simulink model "PIDnLQR"  (R2021a)
settings: Solver=VariableStepAuto  StartTime=0.0  StopTime=4500  RelTol=1e-3
values from neighbouring files (symbols this model uses):
  FF = 1/y(end)    [main.m]
  M = c2d(Mcon,Ts,'zoh')    [main.m]
  SYSdaug = ss(Aaug,Baug,Caug,[],Ts)    [main.m]
  Ts = Mrise/15    [main.m]
undefined symbols (not defined in the file or in its folder): Klqr
libraries: pid_lib x1
settings Model: Creator=andre  LastModifiedBy=Nidhin
settings SolverCC: AlgebraicLoopSolver=TrustRegion
settings DebuggingCC: SFMachineParentedDataDiag=warning

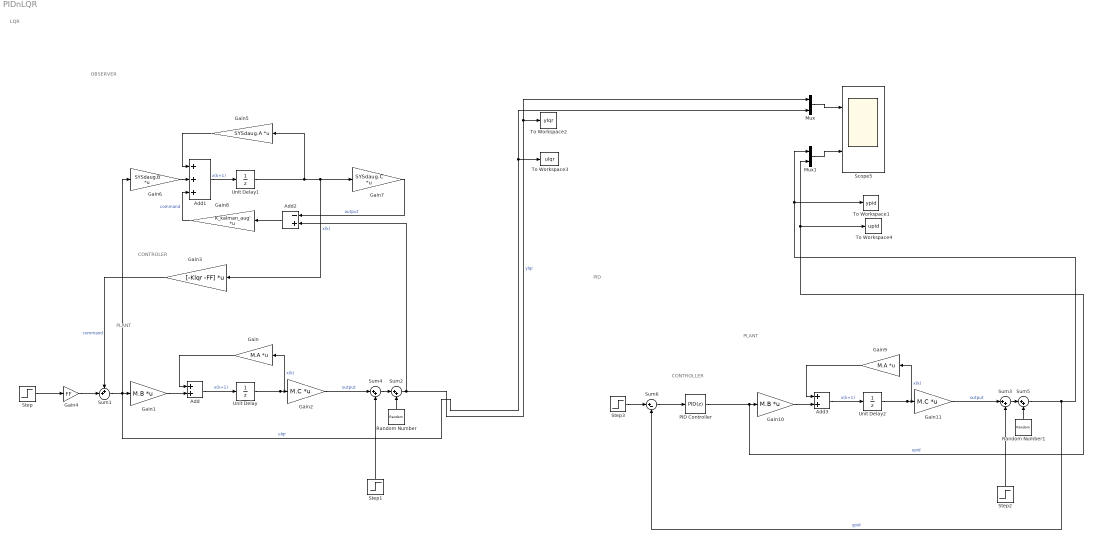
== system PIDnLQR ==
  note: PID
  note: CONTROLLER
  note: CONTROLER
  note: OBSERVER
  note: PLANT
  note: PLANT
  note: LQR
  Add : Sum
  Add1 : Sum  Inputs=+++
  Add2 : Sum  Inputs=-+
  Add3 : Sum
  Gain : Gain  Gain=M.A  Multiplication=Matrix(K*u)
  Gain1 : Gain  Gain=M.B  Multiplication=Matrix(K*u)
  Gain10 : Gain  Gain=M.B  Multiplication=Matrix(K*u)
  Gain11 : Gain  Gain=M.C  Multiplication=Matrix(K*u)
  Gain2 : Gain  Gain=M.C  Multiplication=Matrix(K*u)
  Gain3 : Gain  Gain=[-Klqr -FF]  Multiplication=Matrix(K*u)
  Gain4 : Gain  Gain=FF
  Gain5 : Gain  Gain=SYSdaug.A  Multiplication=Matrix(K*u)
  Gain6 : Gain  Gain=SYSdaug.B  Multiplication=Matrix(K*u)
  Gain7 : Gain  Gain=SYSdaug.C  Multiplication=Matrix(K*u)
  Gain8 : Gain  Gain=K_kalman_aug'  Multiplication=Matrix(K*u)
  Gain9 : Gain  Gain=M.A  Multiplication=Matrix(K*u)
  Mux : Mux  Inputs=2
  Mux1 : Mux  Inputs=2
  PID Controller : pid_lib/PID Controller  Controller=PID  Form=Parallel  TimeDomain=Discrete-time  UseExternalTs=off  SampleTime=Ts  IntegratorMethod=Forward Euler  FilterMethod=Forward Euler  ControllerParametersSource=internal  P=0.051105898923896  I=0.00228966428482342  D=0  UseFilter=on  N=100  TunerSelectOption=Transfer Function Based (PID Tuner App)  InitialConditionSource=internal  InitialConditionForIntegrator=0  InitialConditionForFilter=0  DifferentiatorICPrevScaledInput=0  ExternalReset=none  TrackingMode=off  Kt=1  LimitOutput=off  SatLimitsSource=internal  UpperSaturationLimit=inf  LowerSaturationLimit=-inf  LinearizeAsGain=on  AntiWindupMode=none  Kb=1  POutMin=[]  POutMax=[]  IOutMin=[]  IOutMax=[]  DOutMin=[]  DOutMax=[]  NOutMin=[]  NOutMax=[]  SumOutMin=[]  SumOutMax=[]  SaturationOutMin=[]  SaturationOutMax=[]  PParamMin=[]  PParamMax=[]  IParamMin=[]  IParamMax=[]  DParamMin=[]  DParamMax=[]  NParamMin=[]  NParamMax=[]  KbParamMin=[]  KbParamMax=[]  KtParamMin=[]  KtParamMax=[]  KbOutMin=[]  KbOutMax=[]  KtOutMin=[]  KtOutMax=[]  IntegratorOutMin=[]  IntegratorOutMax=[]  FilterOutMin=[]  FilterOutMax=[]  SumI1OutMin=[]  SumI1OutMax=[]  SumI2OutMin=[]  SumI2OutMax=[]  SumI3OutMin=[]  SumI3OutMax=[]  SumI4OutMin=[]  SumI4OutMax=[]  SumDOutMin=[]  SumDOutMax=[]  DifferentiatorOutMin=[]  DifferentiatorOutMax=[]  FilterDiffOutCoefMin=[]  FilterDiffOutCoefMax=[]  ReciprocalOutMin=[]  ReciprocalOutMax=[]  SumDenOutMin=[]  SumDenOutMax=[]  SumNumOutMin=[]  SumNumOutMax=[]  DivideOutMin=[]  DivideOutMax=[]  UdiffTsProdOutMin=[]  UdiffTsProdOutMax=[]  NTsProdOutMin=[]  NTsProdOutMax=[]  UintegralTsProdOutMin=[]  UintegralTsProdOutMax=[]  UngainTsProdOutMin=[]  UngainTsProdOutMax=[]  IntegratorContinuousStateAttributes=''  IntegratorStateMustResolveToSignalObject=off  IntegratorRTWStateStorageClass=Auto  FilterContinuousStateAttributes=''  FilterStateMustResolveToSignalObject=off  FilterRTWStateStorageClass=Auto  ParallelPVariant=InternalParameters  IdealPVariant=Disabled  IVariant=InternalParameters  DVariant=InternalParameters  IntegratorVariant=Discrete  SatVariant=Disabled  AWVariant=Passthrough  PCopyVariant=Disabled  TRVariant=Disabled  FdbkBlocksVariant=Forward  IdealPFdbkVariant=Disabled  SatFdbkVariant=Disabled  DerivativeFilterVariant=ForwardEulerFilter  NVariant=InternalParameters  NCopyVariant=Disabled  FilterICVariant=InternalICsFilter  IntegratorICVariant=InternalICs  ExternalResetVariant=Disabled  TRSumVariant=Passthrough  SumFdbkVariant=Disabled  SumVariant=Sum_PID  TsampFilterVariant=InternalTs  TsampNgainVariant=Passthrough  TsampIntegralVariant=Passthrough  ExternalSaturationOutDataTypeStr=Inherit: Same as second input
  Random Number : RandomNumber  Variance=0.001  SampleTime=5
  Random Number1 : RandomNumber  Variance=0.001  SampleTime=5
  Scope5 : Scope  NumInputPorts=2
  Step : Step  Time=0  After=3.6  SampleTime=0
  Step1 : Step  Time=50*Ts  After=0.36  SampleTime=0
  Step2 : Step  Time=50*Ts  After=0.36  SampleTime=0
  Step3 : Step  Time=0  After=3.6  SampleTime=0
  Sum1 : Sum  Inputs=++|
  Sum{2..5} (4 alike) : Sum  Inputs=|++
  Sum6 : Sum  Inputs=|+-
  To Workspace1 : ToWorkspace  VariableName=ypid  SaveFormat=Timeseries  SampleTime=-1
  To Workspace2 : ToWorkspace  VariableName=ylqr  SaveFormat=Timeseries  SampleTime=-1
  To Workspace3 : ToWorkspace  VariableName=ulqr  SaveFormat=Timeseries  SampleTime=-1
  To Workspace4 : ToWorkspace  VariableName=upid  SaveFormat=Timeseries  SampleTime=-1
  Unit Delay : UnitDelay  SampleTime=Ts  HasFrameUpgradeWarning=on
  Unit Delay1 : UnitDelay  SampleTime=Ts  HasFrameUpgradeWarning=on
  Unit Delay2 : UnitDelay  SampleTime=Ts  HasFrameUpgradeWarning=on
  wires:
  Gain2/1 -> Sum4/1  "output"
  Add/1 -> Unit Delay/1  "x(k+1)"
  Gain3/1 -> Sum1/1  "command"
  Gain/1 -> Add/1
  Gain1/1 -> Add/2
  Step/1 -> Gain4/1
  Unit Delay/1 -> Gain/1, Gain2/1  "x(k)"
  Unit Delay1/1 -> Gain3/1, Gain7/1, Gain5/1  "x(k)"
  Gain5/1 -> Add1/1
  Gain6/1 -> Add1/2
  Add1/1 -> Unit Delay1/1  "x(k+1)"
  Sum1/1 -> Mux/2, To Workspace3/1, Gain6/1, Gain1/1  "ulqr"
  Gain7/1 -> Add2/1  "output"
  Gain8/1 -> Add1/3  "command"
  Add2/1 -> Gain8/1
  Step1/1 -> Sum4/2
  Sum2/1 -> Add2/2, Mux/1, To Workspace2/1  "ylqr"
  Sum4/1 -> Sum2/1
  Gain4/1 -> Sum1/2
  PID Controller/1 -> Mux1/2, To Workspace4/1, Gain10/1  "upid"
  Gain10/1 -> Add3/2
  Unit Delay2/1 -> Gain9/1, Gain11/1  "x(k)"
  Gain11/1 -> Sum3/1  "output"
  Gain9/1 -> Add3/1
  Add3/1 -> Unit Delay2/1  "x(k+1)"
  Sum3/1 -> Sum5/1
  Random Number1/1 -> Sum5/2
  Sum5/1 -> Sum6/2, To Workspace1/1, Mux1/1  "ypid"
  Sum6/1 -> PID Controller/1
  Step3/1 -> Sum6/1
  Step2/1 -> Sum3/2
  Random Number/1 -> Sum2/2
  Mux/1 -> Scope5/1
  Mux1/1 -> Scope5/2
